simulink model "RenesasCarOnTheTrack"  (R2014a)
settings: Solver=ode3  StartTime=0.0  StopTime=50  FixedStep=1e-3  RelTol=1e-3
values from neighbouring files (symbols this model uses):
  b = 1    [initScript.m]
  left_wheel_speed = 1*10    (= 10)    [initScript.m]
  r = 0.1    [initScript.m]
  right_wheel_speed = right_wheel_speed * (-1)    (= -10)    [initScript.m]
  servo_speed = 0    [initScript.m]
undefined symbols (not defined in the file or in its folder): data, sigbuilder_block, X, Y, Z
libraries: sm_lib x1055, nesl_utility x44, fl_lib x22, simulink x1
(part 5 of 21)

== system RenesasCarOnTheTrack/Renesas_MCU_Car_1_RIGID/x10_1_1_13_RIGID ==
  ReferenceFrame : sm_lib/Frames and Transforms/Reference Frame  BlockFunction=simmechanics.library.frames_transforms.reference_frame
  Solid : sm_lib/Body Elements/Solid  InertiaType=Custom  Mass=0.00026175883509498753  MassUnits=kg  CenterOfMass=[-0.00031902687968783026 0.99992372188601886 6.3655488201488363e-05]  CenterOfMassUnits=mm  MomentsOfInertia=[0.00070957471197172705 0.0011872499998693575 0.00070849613465604996]  MomentsOfInertiaUnits=kg*mm^2  ProductsOfInertia=[-5.3887289074862277e-09 -1.4841649996011424e-07 -3.5037929608807934e-09]  ProductsOfInertiaUnits=kg*mm^2  DensityBased=on  Density=1000  DensityUnits=kg/(m^3)  GraphicType=FromGeometry  MarkerShape=Sphere  MarkerSize=10  MarkerSizeUnits=m  GraphicVisPropType=SimpleVisualProperties  GraphicDiffuseColor=[0.77647058823529413 0.75686274509803919 0.73725490196078436]  GraphicSpecularColor=[0.5 0.5 0.5 1.0]  GraphicAmbientColor=[0.15 0.15 0.15 1.0]  GraphicEmissiveColor=[0.0 0.0 0.0 1.0]  GraphicShininess=75  GraphicOpacity=1  GeometryShape=FromFile  RectangleSize=[1 1]  RectangleSizeUnits=m  BrickDimensions=[1 1 1]  BrickDimensionUnits=m  CylinderRadius=1  CylinderRadiusUnits=m  CylinderLength=1  CylinderLengthUnits=m  SphereRadius=1  SphereRadiusUnits=m  EllipsoidRadii=[1 1 1]  EllipsoidRadiiUnits=m  ExtrusionCrossSection=[1 1; -1 1; -1 -1; 1 -1]  ExtrusionCrossSectionUnits=m  ExtrusionLength=1  ExtrusionLengthUnits=m  PolygonNumSides=3  PolygonOuterRadius=1  PolygonOuterRadiusUnits=m  ExtGeomFileType=STL  ExtGeomFileName=10-1-1_Default_sldprt.STL  ExtGeomFileUnits=mm  RevolutionCrossSection=[1 1; 1 -1; 2 -1; 2 1]  RevolutionCrossSectionUnits=m  RevolutionExtent=Full  RevolutionAngle=180  RevolutionAngleUnits=deg  BlockFunction=simmechanics.library.body_elements.solid
  F : PMIOPort  Port=1  Side=Left
  connections:
  Solid/RConn1 -- ReferenceFrame/RConn1 -- F/RConn1

== system RenesasCarOnTheTrack/Renesas_MCU_Car_1_RIGID/x10_1_1_14_RIGID ==
  ReferenceFrame : sm_lib/Frames and Transforms/Reference Frame  BlockFunction=simmechanics.library.frames_transforms.reference_frame
  Solid : sm_lib/Body Elements/Solid  InertiaType=Custom  Mass=0.00026175883509498753  MassUnits=kg  CenterOfMass=[-0.00031902687968783026 0.99992372188601886 6.3655488201488363e-05]  CenterOfMassUnits=mm  MomentsOfInertia=[0.00070957471197172705 0.0011872499998693575 0.00070849613465604996]  MomentsOfInertiaUnits=kg*mm^2  ProductsOfInertia=[-5.3887289074862277e-09 -1.4841649996011424e-07 -3.5037929608807934e-09]  ProductsOfInertiaUnits=kg*mm^2  DensityBased=on  Density=1000  DensityUnits=kg/(m^3)  GraphicType=FromGeometry  MarkerShape=Sphere  MarkerSize=10  MarkerSizeUnits=m  GraphicVisPropType=SimpleVisualProperties  GraphicDiffuseColor=[0.77647058823529413 0.75686274509803919 0.73725490196078436]  GraphicSpecularColor=[0.5 0.5 0.5 1.0]  GraphicAmbientColor=[0.15 0.15 0.15 1.0]  GraphicEmissiveColor=[0.0 0.0 0.0 1.0]  GraphicShininess=75  GraphicOpacity=1  GeometryShape=FromFile  RectangleSize=[1 1]  RectangleSizeUnits=m  BrickDimensions=[1 1 1]  BrickDimensionUnits=m  CylinderRadius=1  CylinderRadiusUnits=m  CylinderLength=1  CylinderLengthUnits=m  SphereRadius=1  SphereRadiusUnits=m  EllipsoidRadii=[1 1 1]  EllipsoidRadiiUnits=m  ExtrusionCrossSection=[1 1; -1 1; -1 -1; 1 -1]  ExtrusionCrossSectionUnits=m  ExtrusionLength=1  ExtrusionLengthUnits=m  PolygonNumSides=3  PolygonOuterRadius=1  PolygonOuterRadiusUnits=m  ExtGeomFileType=STL  ExtGeomFileName=10-1-1_Default_sldprt.STL  ExtGeomFileUnits=mm  RevolutionCrossSection=[1 1; 1 -1; 2 -1; 2 1]  RevolutionCrossSectionUnits=m  RevolutionExtent=Full  RevolutionAngle=180  RevolutionAngleUnits=deg  BlockFunction=simmechanics.library.body_elements.solid
  F : PMIOPort  Port=1  Side=Left
  connections:
  Solid/RConn1 -- ReferenceFrame/RConn1 -- F/RConn1

== system RenesasCarOnTheTrack/Renesas_MCU_Car_1_RIGID/x10_1_1_15_RIGID ==
  ReferenceFrame : sm_lib/Frames and Transforms/Reference Frame  BlockFunction=simmechanics.library.frames_transforms.reference_frame
  Solid : sm_lib/Body Elements/Solid  InertiaType=Custom  Mass=0.00026175883509498753  MassUnits=kg  CenterOfMass=[-0.00031902687968783026 0.99992372188601886 6.3655488201488363e-05]  CenterOfMassUnits=mm  MomentsOfInertia=[0.00070957471197172705 0.0011872499998693575 0.00070849613465604996]  MomentsOfInertiaUnits=kg*mm^2  ProductsOfInertia=[-5.3887289074862277e-09 -1.4841649996011424e-07 -3.5037929608807934e-09]  ProductsOfInertiaUnits=kg*mm^2  DensityBased=on  Density=1000  DensityUnits=kg/(m^3)  GraphicType=FromGeometry  MarkerShape=Sphere  MarkerSize=10  MarkerSizeUnits=m  GraphicVisPropType=SimpleVisualProperties  GraphicDiffuseColor=[0.77647058823529413 0.75686274509803919 0.73725490196078436]  GraphicSpecularColor=[0.5 0.5 0.5 1.0]  GraphicAmbientColor=[0.15 0.15 0.15 1.0]  GraphicEmissiveColor=[0.0 0.0 0.0 1.0]  GraphicShininess=75  GraphicOpacity=1  GeometryShape=FromFile  RectangleSize=[1 1]  RectangleSizeUnits=m  BrickDimensions=[1 1 1]  BrickDimensionUnits=m  CylinderRadius=1  CylinderRadiusUnits=m  CylinderLength=1  CylinderLengthUnits=m  SphereRadius=1  SphereRadiusUnits=m  EllipsoidRadii=[1 1 1]  EllipsoidRadiiUnits=m  ExtrusionCrossSection=[1 1; -1 1; -1 -1; 1 -1]  ExtrusionCrossSectionUnits=m  ExtrusionLength=1  ExtrusionLengthUnits=m  PolygonNumSides=3  PolygonOuterRadius=1  PolygonOuterRadiusUnits=m  ExtGeomFileType=STL  ExtGeomFileName=10-1-1_Default_sldprt.STL  ExtGeomFileUnits=mm  RevolutionCrossSection=[1 1; 1 -1; 2 -1; 2 1]  RevolutionCrossSectionUnits=m  RevolutionExtent=Full  RevolutionAngle=180  RevolutionAngleUnits=deg  BlockFunction=simmechanics.library.body_elements.solid
  F : PMIOPort  Port=1  Side=Left
  connections:
  Solid/RConn1 -- ReferenceFrame/RConn1 -- F/RConn1

== system RenesasCarOnTheTrack/Renesas_MCU_Car_1_RIGID/x10_1_1_16_RIGID ==
  ReferenceFrame : sm_lib/Frames and Transforms/Reference Frame  BlockFunction=simmechanics.library.frames_transforms.reference_frame
  Solid : sm_lib/Body Elements/Solid  InertiaType=Custom  Mass=0.00026175883509498753  MassUnits=kg  CenterOfMass=[-0.00031902687968783026 0.99992372188601886 6.3655488201488363e-05]  CenterOfMassUnits=mm  MomentsOfInertia=[0.00070957471197172705 0.0011872499998693575 0.00070849613465604996]  MomentsOfInertiaUnits=kg*mm^2  ProductsOfInertia=[-5.3887289074862277e-09 -1.4841649996011424e-07 -3.5037929608807934e-09]  ProductsOfInertiaUnits=kg*mm^2  DensityBased=on  Density=1000  DensityUnits=kg/(m^3)  GraphicType=FromGeometry  MarkerShape=Sphere  MarkerSize=10  MarkerSizeUnits=m  GraphicVisPropType=SimpleVisualProperties  GraphicDiffuseColor=[0.77647058823529413 0.75686274509803919 0.73725490196078436]  GraphicSpecularColor=[0.5 0.5 0.5 1.0]  GraphicAmbientColor=[0.15 0.15 0.15 1.0]  GraphicEmissiveColor=[0.0 0.0 0.0 1.0]  GraphicShininess=75  GraphicOpacity=1  GeometryShape=FromFile  RectangleSize=[1 1]  RectangleSizeUnits=m  BrickDimensions=[1 1 1]  BrickDimensionUnits=m  CylinderRadius=1  CylinderRadiusUnits=m  CylinderLength=1  CylinderLengthUnits=m  SphereRadius=1  SphereRadiusUnits=m  EllipsoidRadii=[1 1 1]  EllipsoidRadiiUnits=m  ExtrusionCrossSection=[1 1; -1 1; -1 -1; 1 -1]  ExtrusionCrossSectionUnits=m  ExtrusionLength=1  ExtrusionLengthUnits=m  PolygonNumSides=3  PolygonOuterRadius=1  PolygonOuterRadiusUnits=m  ExtGeomFileType=STL  ExtGeomFileName=10-1-1_Default_sldprt.STL  ExtGeomFileUnits=mm  RevolutionCrossSection=[1 1; 1 -1; 2 -1; 2 1]  RevolutionCrossSectionUnits=m  RevolutionExtent=Full  RevolutionAngle=180  RevolutionAngleUnits=deg  BlockFunction=simmechanics.library.body_elements.solid
  F : PMIOPort  Port=1  Side=Left
  connections:
  Solid/RConn1 -- ReferenceFrame/RConn1 -- F/RConn1

== system RenesasCarOnTheTrack/Renesas_MCU_Car_1_RIGID/x10_1_1_5_RIGID ==
  ReferenceFrame : sm_lib/Frames and Transforms/Reference Frame  BlockFunction=simmechanics.library.frames_transforms.reference_frame
  Solid : sm_lib/Body Elements/Solid  InertiaType=Custom  Mass=0.00026175883509498753  MassUnits=kg  CenterOfMass=[-0.00031902687968783026 0.99992372188601886 6.3655488201488363e-05]  CenterOfMassUnits=mm  MomentsOfInertia=[0.00070957471197172705 0.0011872499998693575 0.00070849613465604996]  MomentsOfInertiaUnits=kg*mm^2  ProductsOfInertia=[-5.3887289074862277e-09 -1.4841649996011424e-07 -3.5037929608807934e-09]  ProductsOfInertiaUnits=kg*mm^2  DensityBased=on  Density=1000  DensityUnits=kg/(m^3)  GraphicType=FromGeometry  MarkerShape=Sphere  MarkerSize=10  MarkerSizeUnits=m  GraphicVisPropType=SimpleVisualProperties  GraphicDiffuseColor=[0.77647058823529413 0.75686274509803919 0.73725490196078436]  GraphicSpecularColor=[0.5 0.5 0.5 1.0]  GraphicAmbientColor=[0.15 0.15 0.15 1.0]  GraphicEmissiveColor=[0.0 0.0 0.0 1.0]  GraphicShininess=75  GraphicOpacity=1  GeometryShape=FromFile  RectangleSize=[1 1]  RectangleSizeUnits=m  BrickDimensions=[1 1 1]  BrickDimensionUnits=m  CylinderRadius=1  CylinderRadiusUnits=m  CylinderLength=1  CylinderLengthUnits=m  SphereRadius=1  SphereRadiusUnits=m  EllipsoidRadii=[1 1 1]  EllipsoidRadiiUnits=m  ExtrusionCrossSection=[1 1; -1 1; -1 -1; 1 -1]  ExtrusionCrossSectionUnits=m  ExtrusionLength=1  ExtrusionLengthUnits=m  PolygonNumSides=3  PolygonOuterRadius=1  PolygonOuterRadiusUnits=m  ExtGeomFileType=STL  ExtGeomFileName=10-1-1_Default_sldprt.STL  ExtGeomFileUnits=mm  RevolutionCrossSection=[1 1; 1 -1; 2 -1; 2 1]  RevolutionCrossSectionUnits=m  RevolutionExtent=Full  RevolutionAngle=180  RevolutionAngleUnits=deg  BlockFunction=simmechanics.library.body_elements.solid
  F : PMIOPort  Port=1  Side=Left
  connections:
  Solid/RConn1 -- ReferenceFrame/RConn1 -- F/RConn1

== system RenesasCarOnTheTrack/Renesas_MCU_Car_1_RIGID/x10_1_1_6_RIGID ==
  ReferenceFrame : sm_lib/Frames and Transforms/Reference Frame  BlockFunction=simmechanics.library.frames_transforms.reference_frame
  Solid : sm_lib/Body Elements/Solid  InertiaType=Custom  Mass=0.00026175883509498753  MassUnits=kg  CenterOfMass=[-0.00031902687968783026 0.99992372188601886 6.3655488201488363e-05]  CenterOfMassUnits=mm  MomentsOfInertia=[0.00070957471197172705 0.0011872499998693575 0.00070849613465604996]  MomentsOfInertiaUnits=kg*mm^2  ProductsOfInertia=[-5.3887289074862277e-09 -1.4841649996011424e-07 -3.5037929608807934e-09]  ProductsOfInertiaUnits=kg*mm^2  DensityBased=on  Density=1000  DensityUnits=kg/(m^3)  GraphicType=FromGeometry  MarkerShape=Sphere  MarkerSize=10  MarkerSizeUnits=m  GraphicVisPropType=SimpleVisualProperties  GraphicDiffuseColor=[0.77647058823529413 0.75686274509803919 0.73725490196078436]  GraphicSpecularColor=[0.5 0.5 0.5 1.0]  GraphicAmbientColor=[0.15 0.15 0.15 1.0]  GraphicEmissiveColor=[0.0 0.0 0.0 1.0]  GraphicShininess=75  GraphicOpacity=1  GeometryShape=FromFile  RectangleSize=[1 1]  RectangleSizeUnits=m  BrickDimensions=[1 1 1]  BrickDimensionUnits=m  CylinderRadius=1  CylinderRadiusUnits=m  CylinderLength=1  CylinderLengthUnits=m  SphereRadius=1  SphereRadiusUnits=m  EllipsoidRadii=[1 1 1]  EllipsoidRadiiUnits=m  ExtrusionCrossSection=[1 1; -1 1; -1 -1; 1 -1]  ExtrusionCrossSectionUnits=m  ExtrusionLength=1  ExtrusionLengthUnits=m  PolygonNumSides=3  PolygonOuterRadius=1  PolygonOuterRadiusUnits=m  ExtGeomFileType=STL  ExtGeomFileName=10-1-1_Default_sldprt.STL  ExtGeomFileUnits=mm  RevolutionCrossSection=[1 1; 1 -1; 2 -1; 2 1]  RevolutionCrossSectionUnits=m  RevolutionExtent=Full  RevolutionAngle=180  RevolutionAngleUnits=deg  BlockFunction=simmechanics.library.body_elements.solid
  F : PMIOPort  Port=1  Side=Left
  connections:
  Solid/RConn1 -- ReferenceFrame/RConn1 -- F/RConn1

== system RenesasCarOnTheTrack/Renesas_MCU_Car_1_RIGID/x10_1_1_7_RIGID ==
  ReferenceFrame : sm_lib/Frames and Transforms/Reference Frame  BlockFunction=simmechanics.library.frames_transforms.reference_frame
  Solid : sm_lib/Body Elements/Solid  InertiaType=Custom  Mass=0.00026175883509498753  MassUnits=kg  CenterOfMass=[-0.00031902687968783026 0.99992372188601886 6.3655488201488363e-05]  CenterOfMassUnits=mm  MomentsOfInertia=[0.00070957471197172705 0.0011872499998693575 0.00070849613465604996]  MomentsOfInertiaUnits=kg*mm^2  ProductsOfInertia=[-5.3887289074862277e-09 -1.4841649996011424e-07 -3.5037929608807934e-09]  ProductsOfInertiaUnits=kg*mm^2  DensityBased=on  Density=1000  DensityUnits=kg/(m^3)  GraphicType=FromGeometry  MarkerShape=Sphere  MarkerSize=10  MarkerSizeUnits=m  GraphicVisPropType=SimpleVisualProperties  GraphicDiffuseColor=[0.77647058823529413 0.75686274509803919 0.73725490196078436]  GraphicSpecularColor=[0.5 0.5 0.5 1.0]  GraphicAmbientColor=[0.15 0.15 0.15 1.0]  GraphicEmissiveColor=[0.0 0.0 0.0 1.0]  GraphicShininess=75  GraphicOpacity=1  GeometryShape=FromFile  RectangleSize=[1 1]  RectangleSizeUnits=m  BrickDimensions=[1 1 1]  BrickDimensionUnits=m  CylinderRadius=1  CylinderRadiusUnits=m  CylinderLength=1  CylinderLengthUnits=m  SphereRadius=1  SphereRadiusUnits=m  EllipsoidRadii=[1 1 1]  EllipsoidRadiiUnits=m  ExtrusionCrossSection=[1 1; -1 1; -1 -1; 1 -1]  ExtrusionCrossSectionUnits=m  ExtrusionLength=1  ExtrusionLengthUnits=m  PolygonNumSides=3  PolygonOuterRadius=1  PolygonOuterRadiusUnits=m  ExtGeomFileType=STL  ExtGeomFileName=10-1-1_Default_sldprt.STL  ExtGeomFileUnits=mm  RevolutionCrossSection=[1 1; 1 -1; 2 -1; 2 1]  RevolutionCrossSectionUnits=m  RevolutionExtent=Full  RevolutionAngle=180  RevolutionAngleUnits=deg  BlockFunction=simmechanics.library.body_elements.solid
  F : PMIOPort  Port=1  Side=Left
  connections:
  Solid/RConn1 -- ReferenceFrame/RConn1 -- F/RConn1

== system RenesasCarOnTheTrack/Renesas_MCU_Car_1_RIGID/x10_1_1_8_RIGID ==
  ReferenceFrame : sm_lib/Frames and Transforms/Reference Frame  BlockFunction=simmechanics.library.frames_transforms.reference_frame
  Solid : sm_lib/Body Elements/Solid  InertiaType=Custom  Mass=0.00026175883509498753  MassUnits=kg  CenterOfMass=[-0.00031902687968783026 0.99992372188601886 6.3655488201488363e-05]  CenterOfMassUnits=mm  MomentsOfInertia=[0.00070957471197172705 0.0011872499998693575 0.00070849613465604996]  MomentsOfInertiaUnits=kg*mm^2  ProductsOfInertia=[-5.3887289074862277e-09 -1.4841649996011424e-07 -3.5037929608807934e-09]  ProductsOfInertiaUnits=kg*mm^2  DensityBased=on  Density=1000  DensityUnits=kg/(m^3)  GraphicType=FromGeometry  MarkerShape=Sphere  MarkerSize=10  MarkerSizeUnits=m  GraphicVisPropType=SimpleVisualProperties  GraphicDiffuseColor=[0.77647058823529413 0.75686274509803919 0.73725490196078436]  GraphicSpecularColor=[0.5 0.5 0.5 1.0]  GraphicAmbientColor=[0.15 0.15 0.15 1.0]  GraphicEmissiveColor=[0.0 0.0 0.0 1.0]  GraphicShininess=75  GraphicOpacity=1  GeometryShape=FromFile  RectangleSize=[1 1]  RectangleSizeUnits=m  BrickDimensions=[1 1 1]  BrickDimensionUnits=m  CylinderRadius=1  CylinderRadiusUnits=m  CylinderLength=1  CylinderLengthUnits=m  SphereRadius=1  SphereRadiusUnits=m  EllipsoidRadii=[1 1 1]  EllipsoidRadiiUnits=m  ExtrusionCrossSection=[1 1; -1 1; -1 -1; 1 -1]  ExtrusionCrossSectionUnits=m  ExtrusionLength=1  ExtrusionLengthUnits=m  PolygonNumSides=3  PolygonOuterRadius=1  PolygonOuterRadiusUnits=m  ExtGeomFileType=STL  ExtGeomFileName=10-1-1_Default_sldprt.STL  ExtGeomFileUnits=mm  RevolutionCrossSection=[1 1; 1 -1; 2 -1; 2 1]  RevolutionCrossSectionUnits=m  RevolutionExtent=Full  RevolutionAngle=180  RevolutionAngleUnits=deg  BlockFunction=simmechanics.library.body_elements.solid
  F : PMIOPort  Port=1  Side=Left
  connections:
  Solid/RConn1 -- ReferenceFrame/RConn1 -- F/RConn1

== system RenesasCarOnTheTrack/Renesas_MCU_Car_1_RIGID/x10_1_1_9_RIGID ==
  ReferenceFrame : sm_lib/Frames and Transforms/Reference Frame  BlockFunction=simmechanics.library.frames_transforms.reference_frame
  Solid : sm_lib/Body Elements/Solid  InertiaType=Custom  Mass=0.00026175883509498753  MassUnits=kg  CenterOfMass=[-0.00031902687968783026 0.99992372188601886 6.3655488201488363e-05]  CenterOfMassUnits=mm  MomentsOfInertia=[0.00070957471197172705 0.0011872499998693575 0.00070849613465604996]  MomentsOfInertiaUnits=kg*mm^2  ProductsOfInertia=[-5.3887289074862277e-09 -1.4841649996011424e-07 -3.5037929608807934e-09]  ProductsOfInertiaUnits=kg*mm^2  DensityBased=on  Density=1000  DensityUnits=kg/(m^3)  GraphicType=FromGeometry  MarkerShape=Sphere  MarkerSize=10  MarkerSizeUnits=m  GraphicVisPropType=SimpleVisualProperties  GraphicDiffuseColor=[0.77647058823529413 0.75686274509803919 0.73725490196078436]  GraphicSpecularColor=[0.5 0.5 0.5 1.0]  GraphicAmbientColor=[0.15 0.15 0.15 1.0]  GraphicEmissiveColor=[0.0 0.0 0.0 1.0]  GraphicShininess=75  GraphicOpacity=1  GeometryShape=FromFile  RectangleSize=[1 1]  RectangleSizeUnits=m  BrickDimensions=[1 1 1]  BrickDimensionUnits=m  CylinderRadius=1  CylinderRadiusUnits=m  CylinderLength=1  CylinderLengthUnits=m  SphereRadius=1  SphereRadiusUnits=m  EllipsoidRadii=[1 1 1]  EllipsoidRadiiUnits=m  ExtrusionCrossSection=[1 1; -1 1; -1 -1; 1 -1]  ExtrusionCrossSectionUnits=m  ExtrusionLength=1  ExtrusionLengthUnits=m  PolygonNumSides=3  PolygonOuterRadius=1  PolygonOuterRadiusUnits=m  ExtGeomFileType=STL  ExtGeomFileName=10-1-1_Default_sldprt.STL  ExtGeomFileUnits=mm  RevolutionCrossSection=[1 1; 1 -1; 2 -1; 2 1]  RevolutionCrossSectionUnits=m  RevolutionExtent=Full  RevolutionAngle=180  RevolutionAngleUnits=deg  BlockFunction=simmechanics.library.body_elements.solid
  F : PMIOPort  Port=1  Side=Left
  connections:
  Solid/RConn1 -- ReferenceFrame/RConn1 -- F/RConn1

== matlab function RenesasCarOnTheTrack/Virtual Sensors Subsystem/MATLAB Function ==
  data: x input; z input; rotMat input; xRange output; zRange output; r_range input
function [xRange, zRange] = getVirtualBox(x,z,rotMat, r_range)
%#codegen
%% Dimensions
r_range_m = r_range/1000;
% r_range = 0.5;%Radius of SONAR range in 'm'

yb_f = 0.018; %Shift in Z axis from COM

SensorPos = zeros(8,2);
SensorPosNew = zeros(8,3);
%% FRONT SENSORS
SensorPos(1,:) = [r_range_m(1)*sind(-90), r_range_m(1)*cosd(-90)+yb_f];
SensorPos(8,:) = [r_range_m(8)*sind(90), r_range_m(8)*cosd(90)+yb_f];

%Remaining front sensors
i = 2;
for theta = -50:20:50
    SensorPos(i,:) = [r_range_m(i)*sind(theta), r_range_m(i)*cosd(theta)+yb_f];
    i = i+1;
end

rotZ90 = [1 0 0; 0 1 0; 0 0 1];
%rotZ90 = [0 -1 0; 0 1 0; 0 0 1];
rotMatNew = rotMat * rotZ90;
for i = 1:8
    SensorPosNew(i,:) = (rotMatNew*[SensorPos(i,:)';0] + [x; z;0])';
end

xRange = SensorPosNew(:,1);%Inp(:,1);
zRange = SensorPosNew(:,2);%-Inp(:,2);

Ndecimals = 3;

f = 10.^Ndecimals;
xRange = round(f*xRange)/f*(-1);

f = 10.^Ndecimals;
zRange = round(f*zRange)/f;

== matlab function RenesasCarOnTheTrack/Renesas_MCU_Car_1_RIGID/x1_2_3_1_RIGID/MATLAB Function ==
  data: u input; y output
function y = fcn(u)
    %pause(0.0001);
    y = u * (-1);
end

== stateflow chart RenesasCarOnTheTrack/Control Algorithm ==
  state Modes
    en,du:
    leftMostSensors = [SonarSensors(1)] < SensorRanges(1);
    leftMiddleSensors = [SonarSensors(2:3)] < SensorRanges(2:3);
    rightMiddleSensors = [SonarSensors(6:7)] < SensorRanges(6:7);
    rightMostSensors = [SonarSensors(8) ]< SensorRanges(8);
    state GoStraight
      en,du:
      RightVel = v0;
      LeftVel = v0;
    state TurnLeftTight
      du :
      RightVel = v0;
      LeftVel = -v0+(v0/10);
    state TurnRightTight
      du :
      RightVel = -v0+(v0/10);
      LeftVel = v0;
    state TurnLeftWide
      du :
      RightVel = v0;
      LeftVel = -v0+(v0/3);
    state TurnRightWide
      du:
      RightVel = -v0+(v0/3);
      LeftVel = v0;
    (default) -> GoStraight
    TurnLeftWide -> GoStraight : [all(leftMostSensors<1)]
    GoStraight -> TurnLeftWide [order 4] : [any(leftMostSensors>0)]
    TurnLeftTight -> GoStraight : [all(leftMiddleSensors<1)]
    GoStraight -> TurnLeftTight [order 1] : [any(leftMiddleSensors>0)]
    TurnRightTight -> GoStraight : [all(rightMiddleSensors<1)]
    GoStraight -> TurnRightTight [order 2] : [any(rightMiddleSensors>0)]
    TurnRightWide -> GoStraight : [all(rightMostSensors<1)]
    GoStraight -> TurnRightWide [order 3] : [any(rightMostSensors>0)]
  data: LeftVel output; RightVel output; SonarSensors input; frontSensors local; SensorRanges input; v0 parameter; leftMostSensors local; leftMiddleSensors local; rightMostSensors local; rightMiddleSensors local; lineLost local
